simulink model "CompleteModel"  (R2020a)
settings: Solver=ode45  StartTime=0.0  StopTime=endtime  RelTol=1e-3
values from neighbouring files (symbols this model uses):
  DC =     [DC.mat]
  M_matrix = [2.5 0 0; 0 2.50 0; 0 0 1]    [CompleteModel.m]
  Ref = [0;0;0]    [CompleteModel.m]
  SR =     [SR.mat]
  T_bow = [-11.72 -13.257 7.8134 10.766 -1.0091 0.4332 0]    [CompleteModel.m]
  T_coef_PS = [2E-09 3E-07 0.0003 0]    [CompleteModel.m]
  T_coef_SB = [1e-09 2E-07 0.0004 0]    [CompleteModel.m]
  T_matrix = [1 1 0; 0 0 1; -0.065 0.065 0.35]    [CompleteModel.m]
  TauE = [1;0;0]    [CompleteModel.m]
libraries: simulink x7
settings Model: Creator=31620  LastModifiedBy=31620

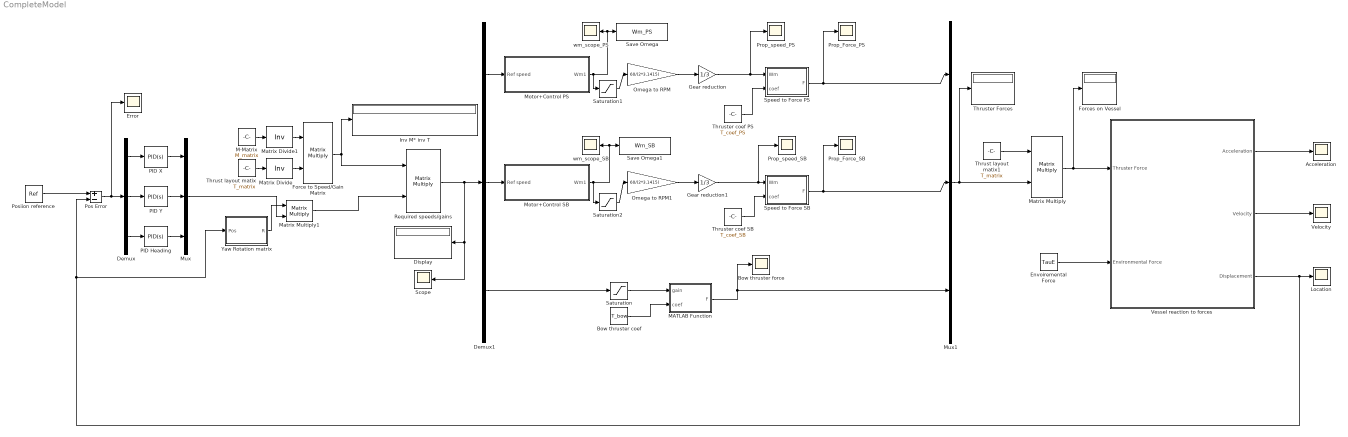
== system CompleteModel ==
  Acceleration : Scope
  Bow thruster coef : Constant  Value=T_bow
  Bow thruster force : Scope
  Demux : Demux  Outputs=3
  Demux1 : Demux  Outputs=3
  Display : Display
  Envoiremental Force : Constant  Value=TauE
  Error : Scope
  Force to Speed/Gain Matrix : Product  Multiplication=Matrix(*)
  Forces on Vessel : Display
  Gear reduction : Gain  Gain=1/3
  Gear reduction1 : Gain  Gain=1/3
  Inv M* inv T : Display
  Location : Scope
  M-Matrix : Constant  Value=M_matrix
  MATLAB Function : MATLAB Function  TreatAsAtomicUnit=on
  Matrix Divide : Product  Inputs=/  Multiplication=Matrix(*)
  Matrix Divide1 : Product  Inputs=/  Multiplication=Matrix(*)
  Matrix Multiply : Product  Multiplication=Matrix(*)
  Matrix Multiply1 : Product  Multiplication=Matrix(*)
  Motor+Control PS : Subsystem
  Motor+Control SB : Subsystem
  Mux : Mux  Inputs=3
  Mux1 : Mux  Inputs=3
  Omega to RPM : Gain  Gain=60/(2*3.1415)
  Omega to RPM1 : Gain  Gain=60/(2*3.1415)
  PID Heading : simulink/Continuous/PID Controller  Controller=PID  Form=Parallel  TimeDomain=Continuous-time  UseExternalTs=off  SampleTime=-1  IntegratorMethod=Forward Euler  FilterMethod=Forward Euler  ControllerParametersSource=internal  P=345.015664616652  I=1.95106877769924  D=7091.38471579827  UseFilter=on  N=7.83169797606647  TunerSelectOption=Transfer Function Based (PID Tuner App)  InitialConditionSource=internal  InitialConditionForIntegrator=0  InitialConditionForFilter=0  DifferentiatorICPrevScaledInput=0  ExternalReset=none  TrackingMode=off  Kt=1  LimitOutput=off  UpperSaturationLimit=inf  LowerSaturationLimit=-inf  LinearizeAsGain=on  AntiWindupMode=none  Kb=1  POutMin=[]  POutMax=[]  IOutMin=[]  IOutMax=[]  DOutMin=[]  DOutMax=[]  NOutMin=[]  NOutMax=[]  SumOutMin=[]  SumOutMax=[]  SaturationOutMin=[]  SaturationOutMax=[]  PParamMin=[]  PParamMax=[]  IParamMin=[]  IParamMax=[]  DParamMin=[]  DParamMax=[]  NParamMin=[]  NParamMax=[]  KbParamMin=[]  KbParamMax=[]  KtParamMin=[]  KtParamMax=[]  KbOutMin=[]  KbOutMax=[]  KtOutMin=[]  KtOutMax=[]  IntegratorOutMin=[]  IntegratorOutMax=[]  FilterOutMin=[]  FilterOutMax=[]  SumI1OutMin=[]  SumI1OutMax=[]  SumI2OutMin=[]  SumI2OutMax=[]  SumI3OutMin=[]  SumI3OutMax=[]  SumI4OutMin=[]  SumI4OutMax=[]  SumDOutMin=[]  SumDOutMax=[]  DifferentiatorOutMin=[]  DifferentiatorOutMax=[]  FilterDiffOutCoefMin=[]  FilterDiffOutCoefMax=[]  ReciprocalOutMin=[]  ReciprocalOutMax=[]  SumDenOutMin=[]  SumDenOutMax=[]  SumNumOutMin=[]  SumNumOutMax=[]  DivideOutMin=[]  DivideOutMax=[]  UdiffTsProdOutMin=[]  UdiffTsProdOutMax=[]  NTsProdOutMin=[]  NTsProdOutMax=[]  UintegralTsProdOutMin=[]  UintegralTsProdOutMax=[]  UngainTsProdOutMin=[]  UngainTsProdOutMax=[]  IntegratorContinuousStateAttributes=''  IntegratorStateMustResolveToSignalObject=off  IntegratorRTWStateStorageClass=Auto  FilterContinuousStateAttributes=''  FilterStateMustResolveToSignalObject=off  FilterRTWStateStorageClass=Auto  ParallelPVariant=InternalParameters  IdealPVariant=Disabled  IVariant=InternalParameters  DVariant=InternalParameters  IntegratorVariant=Continuous  SatVariant=Disabled  AWVariant=Passthrough  PCopyVariant=Disabled  TRVariant=Disabled  FdbkBlocksVariant=Forward  IdealPFdbkVariant=Disabled  SatFdbkVariant=Disabled  DerivativeFilterVariant=ContFilter  NVariant=InternalParameters  NCopyVariant=Disabled  FilterICVariant=InternalICsFilter  IntegratorICVariant=InternalICs  ExternalResetVariant=Disabled  TRSumVariant=Passthrough  SumFdbkVariant=Disabled  SumVariant=Sum_PID  TsampFilterVariant=InternalTs  TsampNgainVariant=Passthrough  TsampIntegralVariant=Passthrough
  PID X : simulink/Continuous/PID Controller  Controller=PID  Form=Ideal  TimeDomain=Continuous-time  UseExternalTs=off  SampleTime=-1  IntegratorMethod=Forward Euler  FilterMethod=Forward Euler  ControllerParametersSource=internal  P=2164.84619235136  I=0.00647665882076123  D=34.3059895929029  UseFilter=on  N=126.873450605204  TunerSelectOption=Transfer Function Based (PID Tuner App)  InitialConditionSource=internal  InitialConditionForIntegrator=0  InitialConditionForFilter=0  DifferentiatorICPrevScaledInput=0  ExternalReset=none  TrackingMode=off  Kt=1  LimitOutput=off  UpperSaturationLimit=inf  LowerSaturationLimit=-inf  LinearizeAsGain=on  AntiWindupMode=none  Kb=1  POutMin=[]  POutMax=[]  IOutMin=[]  IOutMax=[]  DOutMin=[]  DOutMax=[]  NOutMin=[]  NOutMax=[]  SumOutMin=[]  SumOutMax=[]  SaturationOutMin=[]  SaturationOutMax=[]  PParamMin=[]  PParamMax=[]  IParamMin=[]  IParamMax=[]  DParamMin=[]  DParamMax=[]  NParamMin=[]  NParamMax=[]  KbParamMin=[]  KbParamMax=[]  KtParamMin=[]  KtParamMax=[]  KbOutMin=[]  KbOutMax=[]  KtOutMin=[]  KtOutMax=[]  IntegratorOutMin=[]  IntegratorOutMax=[]  FilterOutMin=[]  FilterOutMax=[]  SumI1OutMin=[]  SumI1OutMax=[]  SumI2OutMin=[]  SumI2OutMax=[]  SumI3OutMin=[]  SumI3OutMax=[]  SumI4OutMin=[]  SumI4OutMax=[]  SumDOutMin=[]  SumDOutMax=[]  DifferentiatorOutMin=[]  DifferentiatorOutMax=[]  FilterDiffOutCoefMin=[]  FilterDiffOutCoefMax=[]  ReciprocalOutMin=[]  ReciprocalOutMax=[]  SumDenOutMin=[]  SumDenOutMax=[]  SumNumOutMin=[]  SumNumOutMax=[]  DivideOutMin=[]  DivideOutMax=[]  UdiffTsProdOutMin=[]  UdiffTsProdOutMax=[]  NTsProdOutMin=[]  NTsProdOutMax=[]  UintegralTsProdOutMin=[]  UintegralTsProdOutMax=[]  UngainTsProdOutMin=[]  UngainTsProdOutMax=[]  IntegratorContinuousStateAttributes=''  IntegratorStateMustResolveToSignalObject=off  IntegratorRTWStateStorageClass=Auto  FilterContinuousStateAttributes=''  FilterStateMustResolveToSignalObject=off  FilterRTWStateStorageClass=Auto  ParallelPVariant=Passthrough  IdealPVariant=InternalParameters  IVariant=InternalParameters  DVariant=InternalParameters  IntegratorVariant=Continuous  SatVariant=Disabled  AWVariant=Passthrough  PCopyVariant=Disabled  TRVariant=Disabled  FdbkBlocksVariant=Forward  IdealPFdbkVariant=Disabled  SatFdbkVariant=Disabled  DerivativeFilterVariant=ContFilter  NVariant=InternalParameters  NCopyVariant=Disabled  FilterICVariant=InternalICsFilter  IntegratorICVariant=InternalICs  ExternalResetVariant=Disabled  TRSumVariant=Passthrough  SumFdbkVariant=Disabled  SumVariant=Sum_PID  TsampFilterVariant=InternalTs  TsampNgainVariant=Passthrough  TsampIntegralVariant=Passthrough
  PID Y : simulink/Continuous/PID Controller  Controller=PID  Form=Parallel  TimeDomain=Continuous-time  UseExternalTs=off  SampleTime=-1  IntegratorMethod=Forward Euler  FilterMethod=Forward Euler  ControllerParametersSource=internal  P=310.854605335808  I=9.8955894769747  D=768.887779801729  UseFilter=on  N=454.968011971302  TunerSelectOption=Transfer Function Based (PID Tuner App)  InitialConditionSource=internal  InitialConditionForIntegrator=0  InitialConditionForFilter=0  DifferentiatorICPrevScaledInput=0  ExternalReset=none  TrackingMode=off  Kt=1  LimitOutput=off  UpperSaturationLimit=inf  LowerSaturationLimit=-inf  LinearizeAsGain=on  AntiWindupMode=none  Kb=1  POutMin=[]  POutMax=[]  IOutMin=[]  IOutMax=[]  DOutMin=[]  DOutMax=[]  NOutMin=[]  NOutMax=[]  SumOutMin=[]  SumOutMax=[]  SaturationOutMin=[]  SaturationOutMax=[]  PParamMin=[]  PParamMax=[]  IParamMin=[]  IParamMax=[]  DParamMin=[]  DParamMax=[]  NParamMin=[]  NParamMax=[]  KbParamMin=[]  KbParamMax=[]  KtParamMin=[]  KtParamMax=[]  KbOutMin=[]  KbOutMax=[]  KtOutMin=[]  KtOutMax=[]  IntegratorOutMin=[]  IntegratorOutMax=[]  FilterOutMin=[]  FilterOutMax=[]  SumI1OutMin=[]  SumI1OutMax=[]  SumI2OutMin=[]  SumI2OutMax=[]  SumI3OutMin=[]  SumI3OutMax=[]  SumI4OutMin=[]  SumI4OutMax=[]  SumDOutMin=[]  SumDOutMax=[]  DifferentiatorOutMin=[]  DifferentiatorOutMax=[]  FilterDiffOutCoefMin=[]  FilterDiffOutCoefMax=[]  ReciprocalOutMin=[]  ReciprocalOutMax=[]  SumDenOutMin=[]  SumDenOutMax=[]  SumNumOutMin=[]  SumNumOutMax=[]  DivideOutMin=[]  DivideOutMax=[]  UdiffTsProdOutMin=[]  UdiffTsProdOutMax=[]  NTsProdOutMin=[]  NTsProdOutMax=[]  UintegralTsProdOutMin=[]  UintegralTsProdOutMax=[]  UngainTsProdOutMin=[]  UngainTsProdOutMax=[]  IntegratorContinuousStateAttributes=''  IntegratorStateMustResolveToSignalObject=off  IntegratorRTWStateStorageClass=Auto  FilterContinuousStateAttributes=''  FilterStateMustResolveToSignalObject=off  FilterRTWStateStorageClass=Auto  ParallelPVariant=InternalParameters  IdealPVariant=Disabled  IVariant=InternalParameters  DVariant=InternalParameters  IntegratorVariant=Continuous  SatVariant=Disabled  AWVariant=Passthrough  PCopyVariant=Disabled  TRVariant=Disabled  FdbkBlocksVariant=Forward  IdealPFdbkVariant=Disabled  SatFdbkVariant=Disabled  DerivativeFilterVariant=ContFilter  NVariant=InternalParameters  NCopyVariant=Disabled  FilterICVariant=InternalICsFilter  IntegratorICVariant=InternalICs  ExternalResetVariant=Disabled  TRSumVariant=Passthrough  SumFdbkVariant=Disabled  SumVariant=Sum_PID  TsampFilterVariant=InternalTs  TsampNgainVariant=Passthrough  TsampIntegralVariant=Passthrough
  Pos Error : Sum  Inputs=+-
  Posiion reference : Constant  Value=Ref
  Prop_Force_PS : Scope
  Prop_Force_SB : Scope
  Prop_speed_PS : Scope
  Prop_speed_SB : Scope
  Required speeds/gains : Product  Multiplication=Matrix(*)
  Saturation : Saturate  UpperLimit=0.6  LowerLimit=-0.6
  Saturation1 : Saturate  UpperLimit=1000  LowerLimit=-1000
  Saturation2 : Saturate  UpperLimit=1000  LowerLimit=-1000
  Save Omega : ToWorkspace  VariableName=Wm_PS  SaveFormat=Timeseries  SampleTime=-1
  Save Omega1 : ToWorkspace  VariableName=Wm_SB  SaveFormat=Timeseries  SampleTime=-1
  Scope : Scope
  Speed to Force PS : MATLAB Function  TreatAsAtomicUnit=on
  Speed to Force SB : MATLAB Function  TreatAsAtomicUnit=on
  Thrust layout matix : Constant  Value=T_matrix
  Thrust layout matix1 : Constant  Value=T_matrix
  Thruster Forces : Display
  Thruster coef PS : Constant  Value=T_coef_PS
  Thruster coef SB : Constant  Value=T_coef_SB
  Velocity : Scope
  Vessel reaction to forces : Subsystem
  Yaw Rotation matrix : MATLAB Function  TreatAsAtomicUnit=on
  wm_scope_PS : Scope
  wm_scope_SB : Scope
  wires:
  Envoiremental Force/1 -> Vessel reaction to forces/2(Environmental Force)
  Vessel reaction to forces/1(Acceleration) -> Acceleration/1
  Vessel reaction to forces/2(Velocity) -> Velocity/1
  Vessel reaction to forces/3(Displacement) -> Location/1, Yaw Rotation matrix/1(Pos), Pos Error/2
  Omega to RPM/1 -> Gear reduction/1
  Thruster coef PS/1 -> Speed to Force PS/2(coef)
  Gear reduction/1 -> Prop_speed_PS/1, Speed to Force PS/1(Wm)
  Omega to RPM1/1 -> Gear reduction1/1
  Gear reduction1/1 -> Prop_speed_SB/1, Speed to Force SB/1(Wm)
  Thruster coef SB/1 -> Speed to Force SB/2(coef)
  Speed to Force PS/1(F) -> Prop_Force_PS/1, Mux1/1
  Motor+Control PS/1(Wm1) -> Saturation1/1, wm_scope_PS/1, Save Omega/1
  Motor+Control SB/1(Wm1) -> wm_scope_SB/1, Save Omega1/1, Saturation2/1
  Posiion reference/1 -> Pos Error/1
  Pos Error/1 -> Error/1, Demux/1
  Demux/1 -> PID X/1
  Demux/2 -> PID Y/1
  Demux/3 -> PID Heading/1
  PID Y/1 -> Mux/2
  PID X/1 -> Mux/1
  PID Heading/1 -> Mux/3
  Thrust layout matix/1 -> Matrix Divide/1
  M-Matrix/1 -> Matrix Divide1/1
  Matrix Divide/1 -> Force to Speed/Gain Matrix/2
  Matrix Divide1/1 -> Force to Speed/Gain Matrix/1
  Force to Speed/Gain Matrix/1 -> Required speeds/gains/1, Inv M* inv T/1
  Required speeds/gains/1 -> Scope/1, Display/1, Demux1/1
  Demux1/1 -> Motor+Control PS/1(Ref speed)
  Demux1/2 -> Motor+Control SB/1(Ref speed)
  MATLAB Function/1(F) -> Bow thruster force/1, Mux1/3
  Speed to Force SB/1(F) -> Prop_Force_SB/1, Mux1/2
  Mux1/1 -> Matrix Multiply/2, Thruster Forces/1
  Matrix Multiply/1 -> Forces on Vessel/1, Vessel reaction to forces/1(Thruster Force)
  Thrust layout matix1/1 -> Matrix Multiply/1
  Saturation/1 -> MATLAB Function/1(gain)
  Demux1/3 -> Saturation/1
  Mux/1 -> Matrix Multiply1/2
  Yaw Rotation matrix/1(R) -> Matrix Multiply1/1
  Matrix Multiply1/1 -> Required speeds/gains/2
  Bow thruster coef/1 -> MATLAB Function/2(coef)
  Saturation1/1 -> Omega to RPM/1
  Saturation2/1 -> Omega to RPM1/1

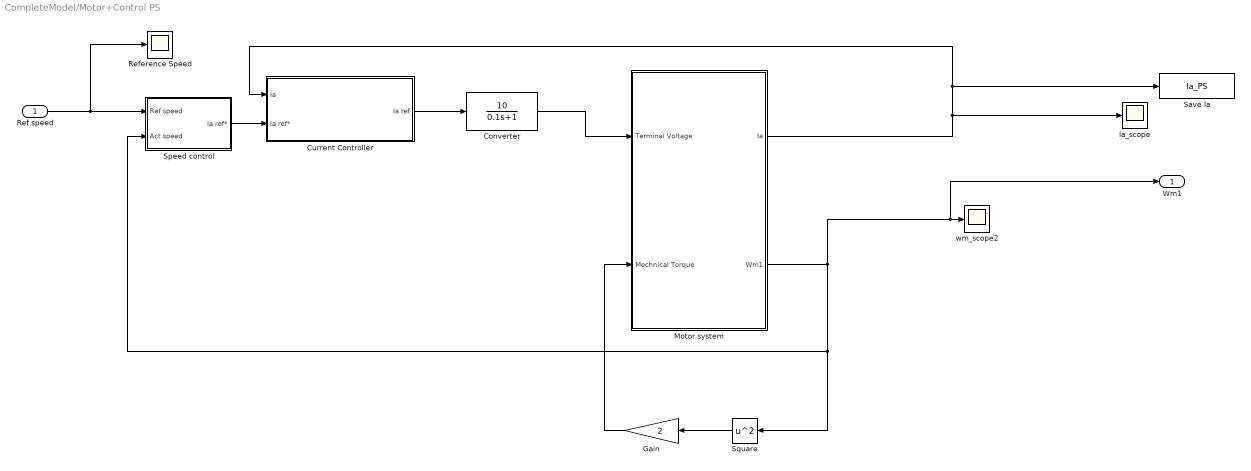
== system CompleteModel/Motor+Control PS ==
  Ref speed : Inport
  Converter : TransferFcn  Numerator=[10]  Denominator=[0.1 1]
  Current Controller : Subsystem
  Gain : Gain  Gain=2
  Ia_scope : Scope
  Motor system : Subsystem
  Reference Speed : Scope
  Save Ia : ToWorkspace  VariableName=Ia_PS  SaveFormat=Timeseries  SampleTime=-1
  Speed control : Subsystem
  Square : Math  Operator=square  SaturateOnIntegerOverflow=on
  wm_scope2 : Scope
  Wm1 : Outport
  wires:
  Gain/1 -> Motor system/2(Mechnical Torque)
  Square/1 -> Gain/1
  Motor system/1(Ia) -> Save Ia/1, Current Controller/1(Ia), Ia_scope/1
  Converter/1 -> Motor system/1(Terminal Voltage)
  Current Controller/1(Ia ref) -> Converter/1
  Motor system/2(Wm1) -> Wm1/1, wm_scope2/1, Square/1, Speed control/2(Act speed)
  Speed control/1(Ia ref*) -> Current Controller/2(Ia ref*)
  Ref speed/1 -> Reference Speed/1, Speed control/1(Ref speed)

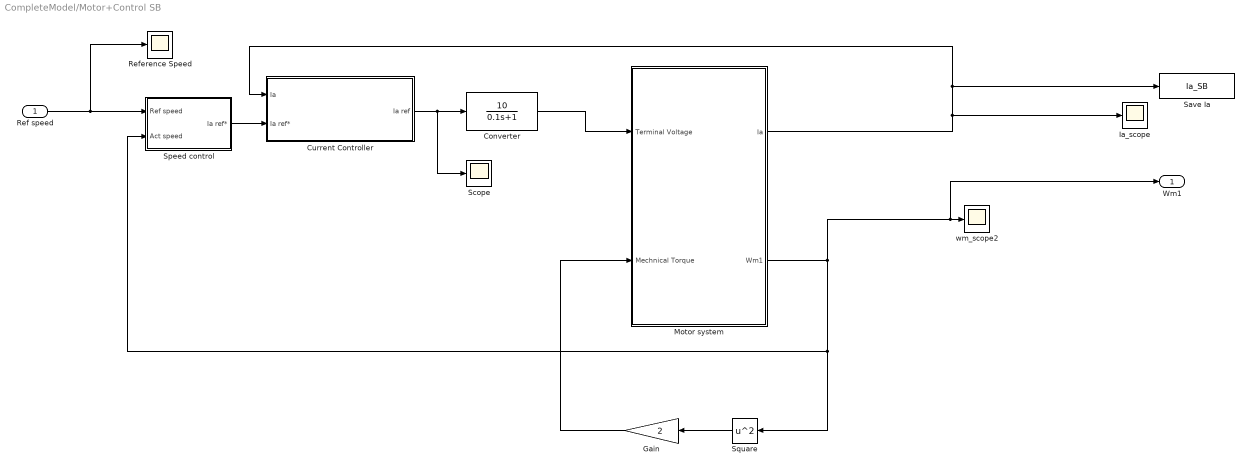
== system CompleteModel/Motor+Control SB ==
  Ref speed : Inport
  Converter : TransferFcn  Numerator=[10]  Denominator=[0.1 1]
  Current Controller : Subsystem
  Gain : Gain  Gain=2
  Ia_scope : Scope
  Motor system : Subsystem
  Reference Speed : Scope
  Save Ia : ToWorkspace  VariableName=Ia_SB  SaveFormat=Timeseries  SampleTime=-1
  Scope : Scope
  Speed control : Subsystem
  Square : Math  Operator=square  SaturateOnIntegerOverflow=on
  wm_scope2 : Scope
  Wm1 : Outport
  wires:
  Gain/1 -> Motor system/2(Mechnical Torque)
  Square/1 -> Gain/1
  Motor system/1(Ia) -> Save Ia/1, Current Controller/1(Ia), Ia_scope/1
  Converter/1 -> Motor system/1(Terminal Voltage)
  Current Controller/1(Ia ref) -> Scope/1, Converter/1
  Motor system/2(Wm1) -> Square/1, Speed control/2(Act speed), Wm1/1, wm_scope2/1
  Speed control/1(Ia ref*) -> Current Controller/2(Ia ref*)
  Ref speed/1 -> Reference Speed/1, Speed control/1(Ref speed)

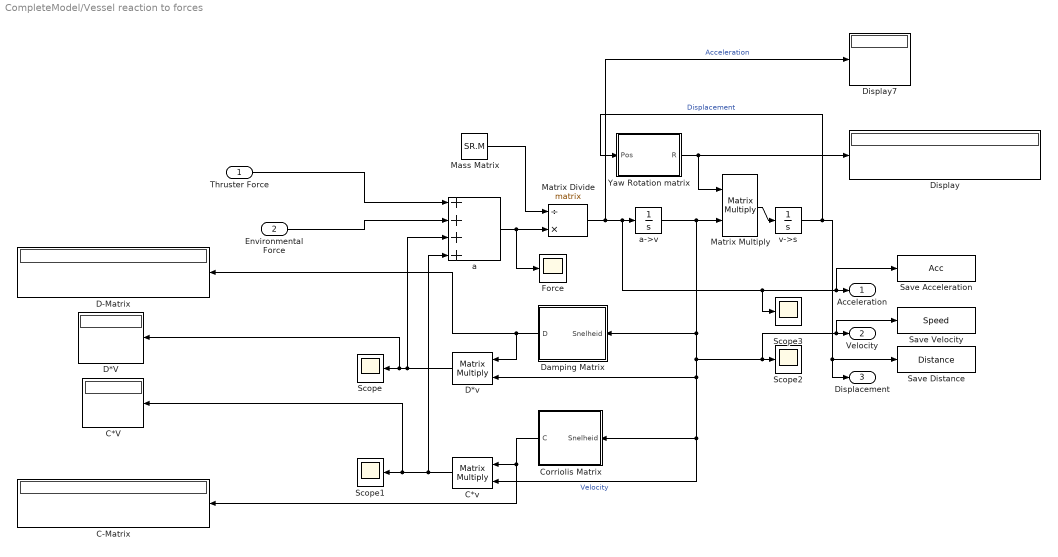
== system CompleteModel/Vessel reaction to forces ==
  Thruster Force : Inport
  Environmental Force : Inport  Port=2
  C*V : Display
  C*v : Product  Multiplication=Matrix(*)
  C-Matrix : Display
  Corriolis Matrix : Subsystem
  D*V : Display
  D*v : Product  Multiplication=Matrix(*)
  D-Matrix : Display
  Damping Matrix : Subsystem
  Display : Display
  Display7 : Display
  Force : Scope
  Mass Matrix : Constant  Value=SR.M
  Matrix Divide : Product  Inputs=/*  Multiplication=Matrix(*)
  Matrix Multiply : Product  Multiplication=Matrix(*)
  Save Acceleration : ToWorkspace  VariableName=Acc  SampleTime=-1
      settings: Decimation=2  Save2DSignal=2-D array (concatenate along first dimension)
  Save Distance : ToWorkspace  VariableName=Distance  SampleTime=-1
      settings: Save2DSignal=2-D array (concatenate along first dimension)
  Save Velocity : ToWorkspace  VariableName=Speed  SampleTime=-1
      settings: Save2DSignal=2-D array (concatenate along first dimension)
  Scope{,1..3} (4 alike) : Scope
  Yaw Rotation matrix : MATLAB Function  TreatAsAtomicUnit=on
  a : Sum  Inputs=++++
  a->v : Integrator
  v->s : Integrator  InitialCondition=[0;0;0]
  Acceleration : Outport
  Velocity : Outport  Port=2
  Displacement : Outport  Port=3
  wires:
  a/1 -> Force/1, Matrix Divide/2
  Corriolis Matrix/1(C) -> C*v/1, C-Matrix/1
  v->s/1 -> Yaw Rotation matrix/1(Pos), Displacement/1, Save Distance/1  "Displacement"
  Damping Matrix/1(D) -> D*v/1, D-Matrix/1
  Environmental Force/1 -> a/2
  Mass Matrix/1 -> Matrix Divide/1
  D*v/1 -> D*V/1, Scope/1, a/3
  C*v/1 -> C*V/1, Scope1/1, a/4
  Yaw Rotation matrix/1(R) -> Matrix Multiply/1, Display/1
  Matrix Multiply/1 -> v->s/1
  Matrix Divide/1 -> Display7/1, Scope3/1, Save Acceleration/1, Acceleration/1, a->v/1  "Acceleration"
  Thruster Force/1 -> a/1
  a->v/1 -> Corriolis Matrix/1(Snelheid), C*v/2, D*v/2, Save Velocity/1, Velocity/1, Scope2/1, Damping Matrix/1(Snelheid), Matrix Multiply/2  "Velocity"

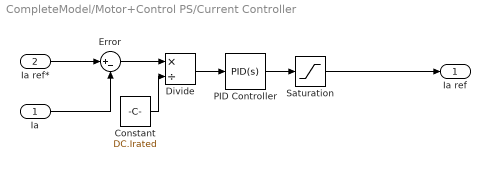
== system CompleteModel/Motor+Control PS/Current Controller ==
  Ia : Inport
  Ia ref* : Inport  Port=2
  Constant : Constant  Value=DC.Irated
  Divide : Product  Inputs=*/
  Error : Sum  Inputs=|+-
  PID Controller : simulink/Continuous/PID Controller  Controller=PID  Form=Ideal  TimeDomain=Continuous-time  UseExternalTs=off  SampleTime=-1  IntegratorMethod=Forward Euler  FilterMethod=Forward Euler  ControllerParametersSource=internal  P=7.2353580328522  I=2.78600690342995  D=0.0824758010540437  UseFilter=on  N=135.726193036092  TunerSelectOption=Transfer Function Based (PID Tuner App)  InitialConditionSource=internal  InitialConditionForIntegrator=0  InitialConditionForFilter=0  DifferentiatorICPrevScaledInput=0  ExternalReset=none  TrackingMode=off  Kt=1  LimitOutput=off  UpperSaturationLimit=inf  LowerSaturationLimit=-inf  LinearizeAsGain=on  AntiWindupMode=none  Kb=1  POutMin=[]  POutMax=[]  IOutMin=[]  IOutMax=[]  DOutMin=[]  DOutMax=[]  NOutMin=[]  NOutMax=[]  SumOutMin=[]  SumOutMax=[]  SaturationOutMin=[]  SaturationOutMax=[]  PParamMin=[]  PParamMax=[]  IParamMin=[]  IParamMax=[]  DParamMin=[]  DParamMax=[]  NParamMin=[]  NParamMax=[]  KbParamMin=[]  KbParamMax=[]  KtParamMin=[]  KtParamMax=[]  KbOutMin=[]  KbOutMax=[]  KtOutMin=[]  KtOutMax=[]  IntegratorOutMin=[]  IntegratorOutMax=[]  FilterOutMin=[]  FilterOutMax=[]  SumI1OutMin=[]  SumI1OutMax=[]  SumI2OutMin=[]  SumI2OutMax=[]  SumI3OutMin=[]  SumI3OutMax=[]  SumI4OutMin=[]  SumI4OutMax=[]  SumDOutMin=[]  SumDOutMax=[]  DifferentiatorOutMin=[]  DifferentiatorOutMax=[]  FilterDiffOutCoefMin=[]  FilterDiffOutCoefMax=[]  ReciprocalOutMin=[]  ReciprocalOutMax=[]  SumDenOutMin=[]  SumDenOutMax=[]  SumNumOutMin=[]  SumNumOutMax=[]  DivideOutMin=[]  DivideOutMax=[]  UdiffTsProdOutMin=[]  UdiffTsProdOutMax=[]  NTsProdOutMin=[]  NTsProdOutMax=[]  UintegralTsProdOutMin=[]  UintegralTsProdOutMax=[]  UngainTsProdOutMin=[]  UngainTsProdOutMax=[]  IntegratorContinuousStateAttributes=''  IntegratorStateMustResolveToSignalObject=off  IntegratorRTWStateStorageClass=Auto  FilterContinuousStateAttributes=''  FilterStateMustResolveToSignalObject=off  FilterRTWStateStorageClass=Auto  ParallelPVariant=Passthrough  IdealPVariant=InternalParameters  IVariant=InternalParameters  DVariant=InternalParameters  IntegratorVariant=Continuous  SatVariant=Disabled  AWVariant=Passthrough  PCopyVariant=Disabled  TRVariant=Disabled  FdbkBlocksVariant=Forward  IdealPFdbkVariant=Disabled  SatFdbkVariant=Disabled  DerivativeFilterVariant=ContFilter  NVariant=InternalParameters  NCopyVariant=Disabled  FilterICVariant=InternalICsFilter  IntegratorICVariant=InternalICs  ExternalResetVariant=Disabled  TRSumVariant=Passthrough  SumFdbkVariant=Disabled  SumVariant=Sum_PID  TsampFilterVariant=InternalTs  TsampNgainVariant=Passthrough  TsampIntegralVariant=Passthrough
  Saturation : Saturate  UpperLimit=1.2*DC.Irated  LowerLimit=-0.5*DC.Irated
  Ia ref : Outport
  wires:
  Error/1 -> Divide/1
  Divide/1 -> PID Controller/1
  PID Controller/1 -> Saturation/1
  Ia/1 -> Error/2
  Saturation/1 -> Ia ref/1
  Ia ref*/1 -> Error/1
  Constant/1 -> Divide/2

== system CompleteModel/Motor+Control PS/Motor system ==
  Terminal Voltage : Inport
  Mechnical Torque : Inport  Port=2
  Electrical Equation : Subsystem
  Mechnical Equation : Subsystem
  Ia : Outport
  Wm1 : Outport  Port=2
  wires:
  Electrical Equation/1(Ia) -> Ia/1, Mechnical Equation/1(Ia)
  Mechnical Torque/1 -> Mechnical Equation/2(Mechnical Torque)
  Terminal Voltage/1 -> Electrical Equation/1(Terminal Voltage)
  Mechnical Equation/1(Wm) -> Wm1/1, Electrical Equation/2(Wm)

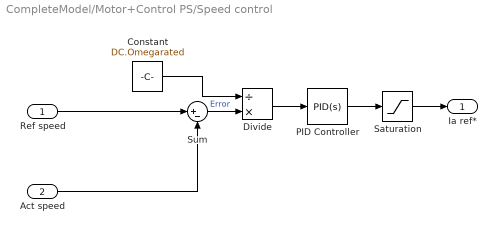
== system CompleteModel/Motor+Control PS/Speed control ==
  Ref speed : Inport
  Act speed : Inport  Port=2
  Constant : Constant  Value=DC.Omegarated
  Divide : Product  Inputs=/*
  PID Controller : simulink/Continuous/PID Controller  Controller=PID  Form=Ideal  TimeDomain=Continuous-time  UseExternalTs=off  SampleTime=-1  IntegratorMethod=Forward Euler  FilterMethod=Forward Euler  ControllerParametersSource=internal  P=16.1905344223384  I=0.203127234448277  D=0.162925883966654  UseFilter=on  N=0.819992914635285  TunerSelectOption=Transfer Function Based (PID Tuner App)  InitialConditionSource=internal  InitialConditionForIntegrator=0  InitialConditionForFilter=0  DifferentiatorICPrevScaledInput=0  ExternalReset=none  TrackingMode=off  Kt=1  LimitOutput=off  UpperSaturationLimit=inf  LowerSaturationLimit=-inf  LinearizeAsGain=on  AntiWindupMode=none  Kb=1  POutMin=[]  POutMax=[]  IOutMin=[]  IOutMax=[]  DOutMin=[]  DOutMax=[]  NOutMin=[]  NOutMax=[]  SumOutMin=[]  SumOutMax=[]  SaturationOutMin=[]  SaturationOutMax=[]  PParamMin=[]  PParamMax=[]  IParamMin=[]  IParamMax=[]  DParamMin=[]  DParamMax=[]  NParamMin=[]  NParamMax=[]  KbParamMin=[]  KbParamMax=[]  KtParamMin=[]  KtParamMax=[]  KbOutMin=[]  KbOutMax=[]  KtOutMin=[]  KtOutMax=[]  IntegratorOutMin=[]  IntegratorOutMax=[]  FilterOutMin=[]  FilterOutMax=[]  SumI1OutMin=[]  SumI1OutMax=[]  SumI2OutMin=[]  SumI2OutMax=[]  SumI3OutMin=[]  SumI3OutMax=[]  SumI4OutMin=[]  SumI4OutMax=[]  SumDOutMin=[]  SumDOutMax=[]  DifferentiatorOutMin=[]  DifferentiatorOutMax=[]  FilterDiffOutCoefMin=[]  FilterDiffOutCoefMax=[]  ReciprocalOutMin=[]  ReciprocalOutMax=[]  SumDenOutMin=[]  SumDenOutMax=[]  SumNumOutMin=[]  SumNumOutMax=[]  DivideOutMin=[]  DivideOutMax=[]  UdiffTsProdOutMin=[]  UdiffTsProdOutMax=[]  NTsProdOutMin=[]  NTsProdOutMax=[]  UintegralTsProdOutMin=[]  UintegralTsProdOutMax=[]  UngainTsProdOutMin=[]  UngainTsProdOutMax=[]  IntegratorContinuousStateAttributes=''  IntegratorStateMustResolveToSignalObject=off  IntegratorRTWStateStorageClass=Auto  FilterContinuousStateAttributes=''  FilterStateMustResolveToSignalObject=off  FilterRTWStateStorageClass=Auto  ParallelPVariant=Passthrough  IdealPVariant=InternalParameters  IVariant=InternalParameters  DVariant=InternalParameters  IntegratorVariant=Continuous  SatVariant=Disabled  AWVariant=Passthrough  PCopyVariant=Disabled  TRVariant=Disabled  FdbkBlocksVariant=Forward  IdealPFdbkVariant=Disabled  SatFdbkVariant=Disabled  DerivativeFilterVariant=ContFilter  NVariant=InternalParameters  NCopyVariant=Disabled  FilterICVariant=InternalICsFilter  IntegratorICVariant=InternalICs  ExternalResetVariant=Disabled  TRSumVariant=Passthrough  SumFdbkVariant=Disabled  SumVariant=Sum_PID  TsampFilterVariant=InternalTs  TsampNgainVariant=Passthrough  TsampIntegralVariant=Passthrough
  Saturation : Saturate  UpperLimit=1.2*DC.Irated  LowerLimit=-0.5*DC.Irated
  Sum : Sum  Inputs=|+-
  Ia ref* : Outport
  wires:
  Saturation/1 -> Ia ref*/1
  PID Controller/1 -> Saturation/1
  Divide/1 -> PID Controller/1
  Ref speed/1 -> Sum/1
  Act speed/1 -> Sum/2
  Sum/1 -> Divide/2  "Error"
  Constant/1 -> Divide/1

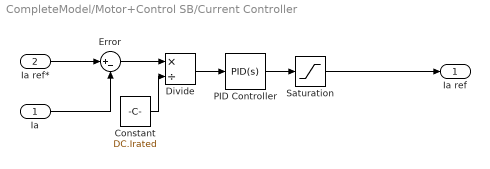
== system CompleteModel/Motor+Control SB/Current Controller ==
  Ia : Inport
  Ia ref* : Inport  Port=2
  Constant : Constant  Value=DC.Irated
  Divide : Product  Inputs=*/
  Error : Sum  Inputs=|+-
  PID Controller : simulink/Continuous/PID Controller  Controller=PID  Form=Ideal  TimeDomain=Continuous-time  UseExternalTs=off  SampleTime=-1  IntegratorMethod=Forward Euler  FilterMethod=Forward Euler  ControllerParametersSource=internal  P=7.2353580328522  I=2.78600690342995  D=0.0824758010540437  UseFilter=on  N=135.726193036092  TunerSelectOption=Transfer Function Based (PID Tuner App)  InitialConditionSource=internal  InitialConditionForIntegrator=0  InitialConditionForFilter=0  DifferentiatorICPrevScaledInput=0  ExternalReset=none  TrackingMode=off  Kt=1  LimitOutput=off  UpperSaturationLimit=inf  LowerSaturationLimit=-inf  LinearizeAsGain=on  AntiWindupMode=none  Kb=1  POutMin=[]  POutMax=[]  IOutMin=[]  IOutMax=[]  DOutMin=[]  DOutMax=[]  NOutMin=[]  NOutMax=[]  SumOutMin=[]  SumOutMax=[]  SaturationOutMin=[]  SaturationOutMax=[]  PParamMin=[]  PParamMax=[]  IParamMin=[]  IParamMax=[]  DParamMin=[]  DParamMax=[]  NParamMin=[]  NParamMax=[]  KbParamMin=[]  KbParamMax=[]  KtParamMin=[]  KtParamMax=[]  KbOutMin=[]  KbOutMax=[]  KtOutMin=[]  KtOutMax=[]  IntegratorOutMin=[]  IntegratorOutMax=[]  FilterOutMin=[]  FilterOutMax=[]  SumI1OutMin=[]  SumI1OutMax=[]  SumI2OutMin=[]  SumI2OutMax=[]  SumI3OutMin=[]  SumI3OutMax=[]  SumI4OutMin=[]  SumI4OutMax=[]  SumDOutMin=[]  SumDOutMax=[]  DifferentiatorOutMin=[]  DifferentiatorOutMax=[]  FilterDiffOutCoefMin=[]  FilterDiffOutCoefMax=[]  ReciprocalOutMin=[]  ReciprocalOutMax=[]  SumDenOutMin=[]  SumDenOutMax=[]  SumNumOutMin=[]  SumNumOutMax=[]  DivideOutMin=[]  DivideOutMax=[]  UdiffTsProdOutMin=[]  UdiffTsProdOutMax=[]  NTsProdOutMin=[]  NTsProdOutMax=[]  UintegralTsProdOutMin=[]  UintegralTsProdOutMax=[]  UngainTsProdOutMin=[]  UngainTsProdOutMax=[]  IntegratorContinuousStateAttributes=''  IntegratorStateMustResolveToSignalObject=off  IntegratorRTWStateStorageClass=Auto  FilterContinuousStateAttributes=''  FilterStateMustResolveToSignalObject=off  FilterRTWStateStorageClass=Auto  ParallelPVariant=Passthrough  IdealPVariant=InternalParameters  IVariant=InternalParameters  DVariant=InternalParameters  IntegratorVariant=Continuous  SatVariant=Disabled  AWVariant=Passthrough  PCopyVariant=Disabled  TRVariant=Disabled  FdbkBlocksVariant=Forward  IdealPFdbkVariant=Disabled  SatFdbkVariant=Disabled  DerivativeFilterVariant=ContFilter  NVariant=InternalParameters  NCopyVariant=Disabled  FilterICVariant=InternalICsFilter  IntegratorICVariant=InternalICs  ExternalResetVariant=Disabled  TRSumVariant=Passthrough  SumFdbkVariant=Disabled  SumVariant=Sum_PID  TsampFilterVariant=InternalTs  TsampNgainVariant=Passthrough  TsampIntegralVariant=Passthrough
  Saturation : Saturate  UpperLimit=1.2*DC.Irated  LowerLimit=-0.5*DC.Irated
  Ia ref : Outport
  wires:
  Error/1 -> Divide/1
  Divide/1 -> PID Controller/1
  PID Controller/1 -> Saturation/1
  Ia/1 -> Error/2
  Saturation/1 -> Ia ref/1
  Ia ref*/1 -> Error/1
  Constant/1 -> Divide/2

== system CompleteModel/Motor+Control SB/Motor system ==
  Terminal Voltage : Inport
  Mechnical Torque : Inport  Port=2
  Electrical Equation : Subsystem
  Mechnical Equation : Subsystem
  Ia : Outport
  Wm1 : Outport  Port=2
  wires:
  Electrical Equation/1(Ia) -> Ia/1, Mechnical Equation/1(Ia)
  Mechnical Torque/1 -> Mechnical Equation/2(Mechnical Torque)
  Terminal Voltage/1 -> Electrical Equation/1(Terminal Voltage)
  Mechnical Equation/1(Wm) -> Wm1/1, Electrical Equation/2(Wm)

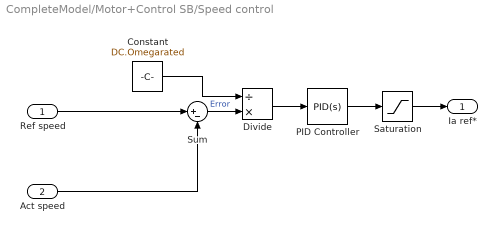
== system CompleteModel/Motor+Control SB/Speed control ==
  Ref speed : Inport
  Act speed : Inport  Port=2
  Constant : Constant  Value=DC.Omegarated
  Divide : Product  Inputs=/*
  PID Controller : simulink/Continuous/PID Controller  Controller=PID  Form=Ideal  TimeDomain=Continuous-time  UseExternalTs=off  SampleTime=-1  IntegratorMethod=Forward Euler  FilterMethod=Forward Euler  ControllerParametersSource=internal  P=16.1905344223384  I=0.203127234448277  D=0.162925883966654  UseFilter=on  N=0.819992914635285  TunerSelectOption=Transfer Function Based (PID Tuner App)  InitialConditionSource=internal  InitialConditionForIntegrator=0  InitialConditionForFilter=0  DifferentiatorICPrevScaledInput=0  ExternalReset=none  TrackingMode=off  Kt=1  LimitOutput=off  UpperSaturationLimit=inf  LowerSaturationLimit=-inf  LinearizeAsGain=on  AntiWindupMode=none  Kb=1  POutMin=[]  POutMax=[]  IOutMin=[]  IOutMax=[]  DOutMin=[]  DOutMax=[]  NOutMin=[]  NOutMax=[]  SumOutMin=[]  SumOutMax=[]  SaturationOutMin=[]  SaturationOutMax=[]  PParamMin=[]  PParamMax=[]  IParamMin=[]  IParamMax=[]  DParamMin=[]  DParamMax=[]  NParamMin=[]  NParamMax=[]  KbParamMin=[]  KbParamMax=[]  KtParamMin=[]  KtParamMax=[]  KbOutMin=[]  KbOutMax=[]  KtOutMin=[]  KtOutMax=[]  IntegratorOutMin=[]  IntegratorOutMax=[]  FilterOutMin=[]  FilterOutMax=[]  SumI1OutMin=[]  SumI1OutMax=[]  SumI2OutMin=[]  SumI2OutMax=[]  SumI3OutMin=[]  SumI3OutMax=[]  SumI4OutMin=[]  SumI4OutMax=[]  SumDOutMin=[]  SumDOutMax=[]  DifferentiatorOutMin=[]  DifferentiatorOutMax=[]  FilterDiffOutCoefMin=[]  FilterDiffOutCoefMax=[]  ReciprocalOutMin=[]  ReciprocalOutMax=[]  SumDenOutMin=[]  SumDenOutMax=[]  SumNumOutMin=[]  SumNumOutMax=[]  DivideOutMin=[]  DivideOutMax=[]  UdiffTsProdOutMin=[]  UdiffTsProdOutMax=[]  NTsProdOutMin=[]  NTsProdOutMax=[]  UintegralTsProdOutMin=[]  UintegralTsProdOutMax=[]  UngainTsProdOutMin=[]  UngainTsProdOutMax=[]  IntegratorContinuousStateAttributes=''  IntegratorStateMustResolveToSignalObject=off  IntegratorRTWStateStorageClass=Auto  FilterContinuousStateAttributes=''  FilterStateMustResolveToSignalObject=off  FilterRTWStateStorageClass=Auto  ParallelPVariant=Passthrough  IdealPVariant=InternalParameters  IVariant=InternalParameters  DVariant=InternalParameters  IntegratorVariant=Continuous  SatVariant=Disabled  AWVariant=Passthrough  PCopyVariant=Disabled  TRVariant=Disabled  FdbkBlocksVariant=Forward  IdealPFdbkVariant=Disabled  SatFdbkVariant=Disabled  DerivativeFilterVariant=ContFilter  NVariant=InternalParameters  NCopyVariant=Disabled  FilterICVariant=InternalICsFilter  IntegratorICVariant=InternalICs  ExternalResetVariant=Disabled  TRSumVariant=Passthrough  SumFdbkVariant=Disabled  SumVariant=Sum_PID  TsampFilterVariant=InternalTs  TsampNgainVariant=Passthrough  TsampIntegralVariant=Passthrough
  Saturation : Saturate  UpperLimit=1.2*DC.Irated  LowerLimit=-0.5*DC.Irated
  Sum : Sum  Inputs=|+-
  Ia ref* : Outport
  wires:
  Saturation/1 -> Ia ref*/1
  PID Controller/1 -> Saturation/1
  Divide/1 -> PID Controller/1
  Ref speed/1 -> Sum/1
  Act speed/1 -> Sum/2
  Sum/1 -> Divide/2  "Error"
  Constant/1 -> Divide/1

== system CompleteModel/Vessel reaction to forces/Corriolis Matrix ==
  Snelheid : Inport
  MATLAB Function1 : MATLAB Function  TreatAsAtomicUnit=on
  Mass : Constant  Value=SR.m
  Xudot : Constant  Value=SR.Xudot
  Yvdot : Constant  Value=SR.Yvdot
  C : Outport
  wires:
  Yvdot/1 -> MATLAB Function1/3(Yvdot)
  MATLAB Function1/1(C) -> C/1
  Xudot/1 -> MATLAB Function1/2(Xudot)
  Mass/1 -> MATLAB Function1/4(m)
  Snelheid/1 -> MATLAB Function1/1(uv)

== system CompleteModel/Vessel reaction to forces/Damping Matrix ==
  Snelheid : Inport
  Damping : MATLAB Function  TreatAsAtomicUnit=on
  Length : Constant  Value=SR.L
  Xdrag_coef : Constant  Value=SR.Xdrag_coef
  Yaw_coef : Constant  Value=SR.Yaw_coef
  Ydrag_coef : Constant  Value=SR.Ydrag_coef
  D : Outport
  wires:
  Length/1 -> Damping/5(L)
  Ydrag_coef/1 -> Damping/3(Y)
  Yaw_coef/1 -> Damping/4(Yaw)
  Xdrag_coef/1 -> Damping/2(X)
  Snelheid/1 -> Damping/1(uvr)
  Damping/1(D) -> D/1

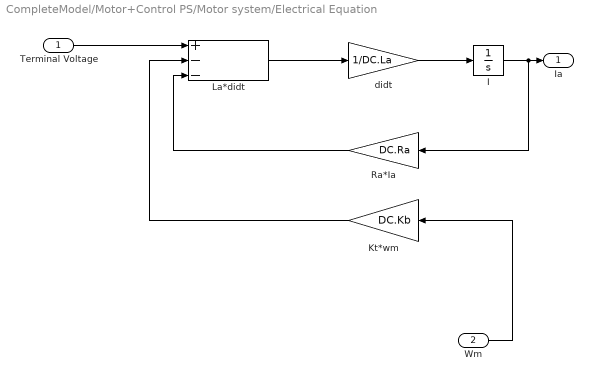
== system CompleteModel/Motor+Control PS/Motor system/Electrical Equation ==
  Terminal Voltage : Inport
  Wm : Inport  Port=2
  I : Integrator
  Kt*wm : Gain  Gain=DC.Kb
  La*didt : Sum  Inputs=+--
  Ra*Ia : Gain  Gain=DC.Ra
  didt : Gain  Gain=1/DC.La
  Ia : Outport
  wires:
  Wm/1 -> Kt*wm/1
  Kt*wm/1 -> La*didt/2
  didt/1 -> I/1
  Terminal Voltage/1 -> La*didt/1
  La*didt/1 -> didt/1
  Ra*Ia/1 -> La*didt/3
  I/1 -> Ra*Ia/1, Ia/1

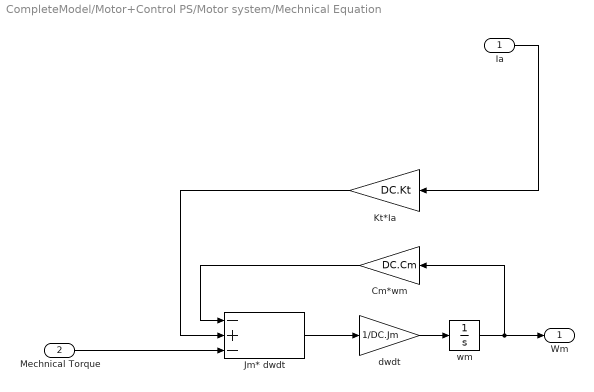
== system CompleteModel/Motor+Control PS/Motor system/Mechnical Equation ==
  Ia : Inport
  Mechnical Torque : Inport  Port=2
  Cm*wm : Gain  Gain=DC.Cm
  Jm* dwdt : Sum  Inputs=-+-
  Kt*Ia : Gain  Gain=DC.Kt
  dwdt : Gain  Gain=1/DC.Jm
  wm : Integrator
  Wm : Outport
  wires:
  wm/1 -> Cm*wm/1, Wm/1
  dwdt/1 -> wm/1
  Mechnical Torque/1 -> Jm* dwdt/3
  Cm*wm/1 -> Jm* dwdt/1
  Jm* dwdt/1 -> dwdt/1
  Ia/1 -> Kt*Ia/1
  Kt*Ia/1 -> Jm* dwdt/2

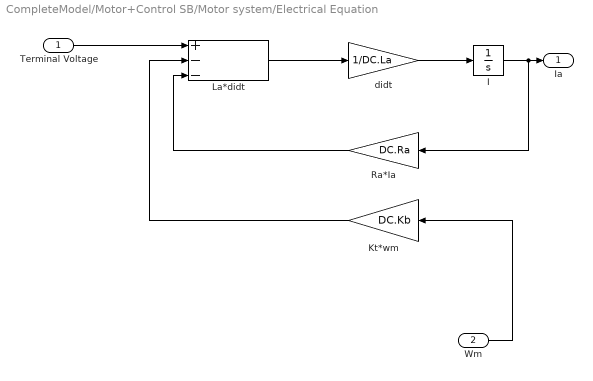
== system CompleteModel/Motor+Control SB/Motor system/Electrical Equation ==
  Terminal Voltage : Inport
  Wm : Inport  Port=2
  I : Integrator
  Kt*wm : Gain  Gain=DC.Kb
  La*didt : Sum  Inputs=+--
  Ra*Ia : Gain  Gain=DC.Ra
  didt : Gain  Gain=1/DC.La
  Ia : Outport
  wires:
  Wm/1 -> Kt*wm/1
  Kt*wm/1 -> La*didt/2
  didt/1 -> I/1
  Terminal Voltage/1 -> La*didt/1
  La*didt/1 -> didt/1
  Ra*Ia/1 -> La*didt/3
  I/1 -> Ra*Ia/1, Ia/1

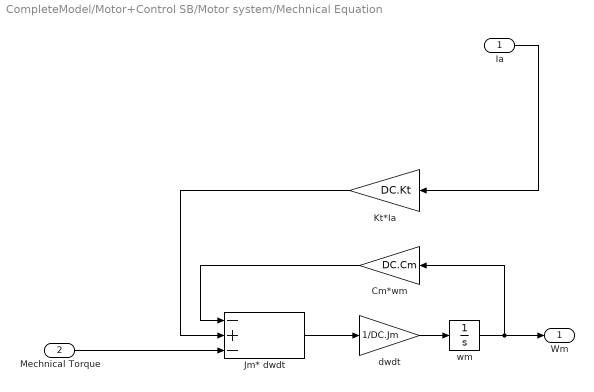
== system CompleteModel/Motor+Control SB/Motor system/Mechnical Equation ==
  Ia : Inport
  Mechnical Torque : Inport  Port=2
  Cm*wm : Gain  Gain=DC.Cm
  Jm* dwdt : Sum  Inputs=-+-
  Kt*Ia : Gain  Gain=DC.Kt
  dwdt : Gain  Gain=1/DC.Jm
  wm : Integrator
  Wm : Outport
  wires:
  wm/1 -> Cm*wm/1, Wm/1
  dwdt/1 -> wm/1
  Mechnical Torque/1 -> Jm* dwdt/3
  Cm*wm/1 -> Jm* dwdt/1
  Jm* dwdt/1 -> dwdt/1
  Ia/1 -> Kt*Ia/1
  Kt*Ia/1 -> Jm* dwdt/2

== matlab function CompleteModel/Vessel reaction to forces/Corriolis Matrix/MATLAB Function1 ==
  data: uv input; C output; Xudot input; Yvdot input; m input
function C = fcn(uv, Xudot, Yvdot, m)
a1 = Xudot*uv(1)+0*uv(2);
a2 = 0*uv(1)+Yvdot*uv(2);

Ca = [0 0 a2; 0 0 -a1; -a2 a1 0];

Crb = [0 0 -m*uv(2); 0 0 m*uv(1); m*uv(2) -m*uv(1) 0];

C = Ca+Crb;

== matlab function CompleteModel/Vessel reaction to forces/Damping Matrix/Damping ==
  data: uvr input; D output; X input; Y input; Yaw input; L input
function D = fcn(uvr, X, Y, Yaw, L)
    D11 = X(1)*uvr(1)^3+X(2)*uvr(1)^2+X(3)*uvr(1)+X(4);
    D22 = Y(1)*uvr(2)^2+Y(2)*uvr(2)^2+Y(3)*uvr(2)+Y(4);
    D33 = 1/80*Yaw(1)*uvr(3)^2*L^4+1/12*Yaw(2)*L^2;
D = [D11 0 0; 0 D22 0; 0 0 D33];

== matlab function CompleteModel/Speed to Force PS ==
  data: Wm input; F output; coef input
function F = fcn(Wm, coef)

F = coef(1)*Wm^3+coef(2)*Wm^2+coef(3)*Wm+coef(4);

== matlab function CompleteModel/Speed to Force SB ==
  data: Wm input; F output; coef input
function F = fcn(Wm, coef)

F = coef(1)*Wm^3+coef(2)*Wm^2+coef(3)*Wm+coef(4);

== matlab function CompleteModel/Vessel reaction to forces/Yaw Rotation matrix ==
  data: Pos input; R output
function R = fcn(Pos)
Phi = -Pos(3);
R = [cos(Phi) -sin(Phi) 0; sin(Phi) cos(Phi) 0 ; 0 0 1];

== matlab function CompleteModel/Yaw Rotation matrix ==
  data: Pos input; R output
function R = fcn(Pos)
Phi = -Pos(3);
R = [cos(Phi) -sin(Phi) 0; sin(Phi) cos(Phi) 0 ; 0 0 1];

== matlab function CompleteModel/MATLAB Function ==
  data: gain input; F output; coef input
function F = fcn(gain,coef)

F = coef(1)*gain^6+coef(2)*gain^5+coef(3)*gain^4+coef(4)*gain^3+coef(5)*gain^2+coef(6)*gain+coef(7);
